simulink model "RigidArmModel_2D"  (R2019a)
settings: Solver=VariableStepAuto  StartTime=0.0  StopTime=stopTime  RelTol=1e-3
undefined symbols (not defined in the file): init_theta_1, init_theta_2, init_theta_dot_1, init_theta_dot_2, k1, k2, L1, L2, m1, m2, t1, t2, x_des, y_des
settings Model: Creator=Shaon  LastModifiedBy=Shaon

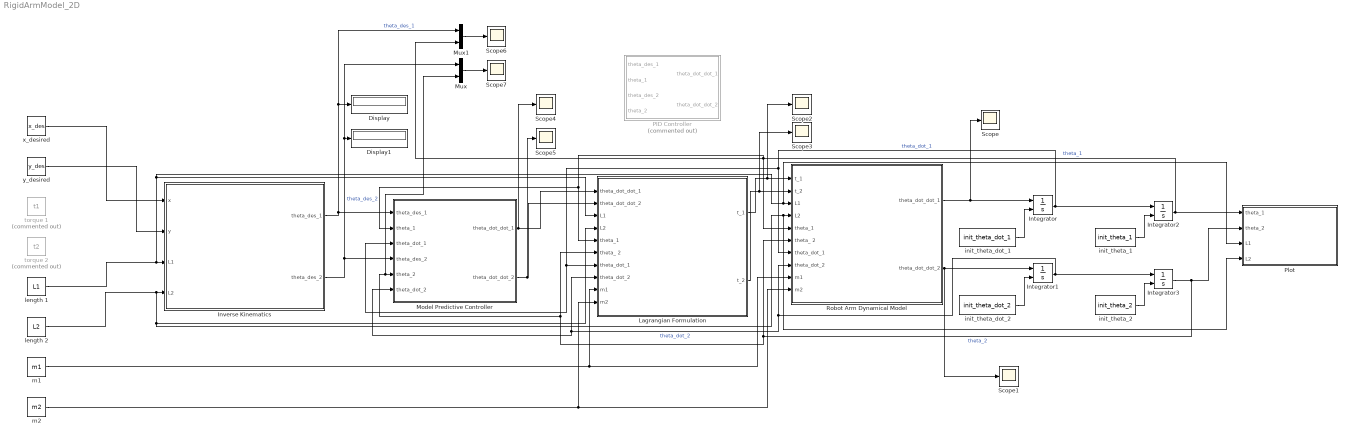
== system RigidArmModel_2D ==
  Display : Display
  Display1 : Display
  Integrator{,1..3} (4 alike) : Integrator  InitialConditionSource=external
  Inverse Kinematics : Subsystem
  Lagrangian Formulation : Subsystem
  Model Predictive Controller : Subsystem
  Mux : Mux  Inputs=2
  Mux1 : Mux  Inputs=2
  PID Controller : Subsystem  Commented=on
  Plot : MATLAB Function  TreatAsAtomicUnit=on
  Robot Arm Dynamical Model : Subsystem
  Scope{,1..7} (8 alike) : Scope
  init_theta_1 : Constant  Value=init_theta_1
  init_theta_2 : Constant  Value=init_theta_2
  init_theta_dot_1 : Constant  Value=init_theta_dot_1
  init_theta_dot_2 : Constant  Value=init_theta_dot_2
  length 1 : Constant  Value=L1
  length 2 : Constant  Value=L2
  m1 : Constant  Value=m1
  m2 : Constant  Value=m2
  torque 1 : Constant  Commented=on  Value=t1
  torque 2 : Constant  Commented=on  Value=t2
  x_desired : Constant  Value=x_des
  y_desired : Constant  Value=y_des
  wires:
  Robot Arm Dynamical Model/1(theta_dot_dot_1) -> Scope/1, Integrator/1
  Robot Arm Dynamical Model/2(theta_dot_dot_2) -> Integrator1/1, Scope1/1
  Integrator/1 -> Robot Arm Dynamical Model/7(theta_dot_1), Model Predictive Controller/3(theta_dot_1), Lagrangian Formulation/7(theta_dot_1), Integrator2/1  "theta_dot_1"
  Integrator1/1 -> Lagrangian Formulation/8(theta_dot_2), Model Predictive Controller/6(theta_dot_2), Robot Arm Dynamical Model/8(theta_dot_2), Integrator3/1  "theta_dot_2"
  Integrator2/1 -> Robot Arm Dynamical Model/5("theta_1 "), Lagrangian Formulation/5("theta_1 "), Model Predictive Controller/2(theta_1), Mux1/2, Plot/1(theta_1)  "theta_1"
  Integrator3/1 -> Lagrangian Formulation/6(theta_ 2), Mux/2, Model Predictive Controller/5(theta_2), Robot Arm Dynamical Model/6(theta_ 2), Plot/2(theta_2)  "theta_2"
  init_theta_1/1 -> Integrator2/2
  init_theta_2/1 -> Integrator3/2
  init_theta_dot_1/1 -> Integrator/2
  init_theta_dot_2/1 -> Integrator1/2
  Inverse Kinematics/1(theta_des_1) -> Model Predictive Controller/1(theta_des_1), Mux1/1, Display/1  "theta_des_1"
  Inverse Kinematics/2(theta_des_2) -> Model Predictive Controller/4(theta_des_2), Mux/1, Display1/1  "theta_des_2"
  x_desired/1 -> Inverse Kinematics/1(x)
  y_desired/1 -> Inverse Kinematics/2(y)
  length 1/1 -> Lagrangian Formulation/3(L1), Plot/3(L1), Robot Arm Dynamical Model/3(L1), Inverse Kinematics/3(L1)
  length 2/1 -> Lagrangian Formulation/4(L2), Plot/4(L2), Robot Arm Dynamical Model/4(L2), Inverse Kinematics/4(L2)
  Lagrangian Formulation/1(t_1) -> Robot Arm Dynamical Model/1(t_1), Scope2/1
  Lagrangian Formulation/2(t_2) -> Robot Arm Dynamical Model/2(t_2), Scope3/1
  m1/1 -> Lagrangian Formulation/9(m1), Robot Arm Dynamical Model/9(m1)
  m2/1 -> Lagrangian Formulation/10(m2), Robot Arm Dynamical Model/10(m2)
  Mux/1 -> Scope7/1
  Mux1/1 -> Scope6/1
  Model Predictive Controller/1(theta_dot_dot_1) -> Scope4/1, Lagrangian Formulation/1(theta_dot_dot_1)
  Model Predictive Controller/2(theta_dot_dot_2) -> Scope5/1, Lagrangian Formulation/2(theta_dot_dot_2)

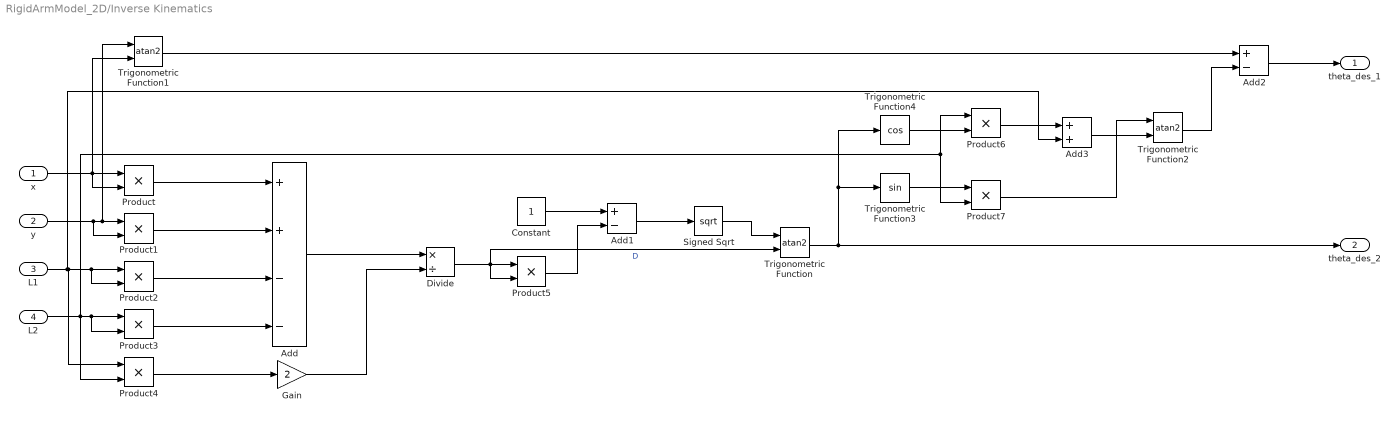
== system RigidArmModel_2D/Inverse Kinematics ==
  x : Inport
  y : Inport  Port=2
  L1 : Inport  Port=3
  L2 : Inport  Port=4
  Add : Sum  Inputs=++--
  Add1 : Sum  Inputs=+-
  Add2 : Sum  Inputs=+-
  Add3 : Sum
  Constant : Constant
  Divide : Product  Inputs=*/
  Gain : Gain  Gain=2
  Product{,1..7} (8 alike) : Product
  Signed Sqrt : Sqrt  SaturateOnIntegerOverflow=on
  Trigonometric Function : Trigonometry  Operator=atan2
  Trigonometric Function1 : Trigonometry  Operator=atan2
  Trigonometric Function2 : Trigonometry  Operator=atan2
  Trigonometric Function3 : Trigonometry
  Trigonometric Function4 : Trigonometry  Operator=cos
  theta_des_1 : Outport
  theta_des_2 : Outport  Port=2
  wires:
  Trigonometric Function2/1 -> Add2/2
  Trigonometric Function/1 -> theta_des_2/1, Trigonometric Function4/1, Trigonometric Function3/1
  Product1/1 -> Add/2
  Product/1 -> Add/1
  Trigonometric Function3/1 -> Product7/1
  y/1 -> Product1/1, Trigonometric Function1/1, Product1/2
  L2/1 -> Product6/1, Product7/2, Product4/2, Product3/2, Product3/1
  Trigonometric Function1/1 -> Add2/1
  Product6/1 -> Add3/1
  Trigonometric Function4/1 -> Product6/2
  Add2/1 -> theta_des_1/1
  Add3/1 -> Trigonometric Function2/2
  Constant/1 -> Add1/1
  L1/1 -> Add3/2, Product4/1, Product2/2, Product2/1
  Signed Sqrt/1 -> Trigonometric Function/1
  Add/1 -> Divide/1
  Product7/1 -> Trigonometric Function2/1
  x/1 -> Product/2, Product/1, Trigonometric Function1/2
  Product5/1 -> Add1/2
  Product2/1 -> Add/3
  Add1/1 -> Signed Sqrt/1
  Divide/1 -> Product5/2, Product5/1, Trigonometric Function/2  "D"
  Gain/1 -> Divide/2
  Product4/1 -> Gain/1
  Product3/1 -> Add/4

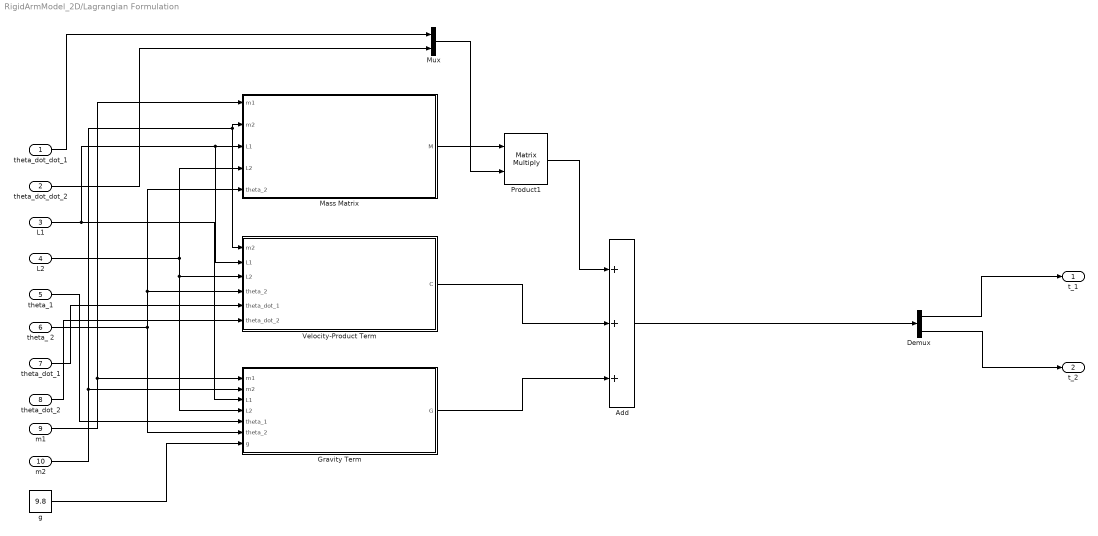
== system RigidArmModel_2D/Lagrangian Formulation ==
  theta_dot_dot_1 : Inport
  theta_dot_dot_2 : Inport  Port=2
  L1 : Inport  Port=3
  L2 : Inport  Port=4
  "theta_1 " : Inport  Port=5
  theta_ 2 : Inport  Port=6
  theta_dot_1 : Inport  Port=7
  theta_dot_2 : Inport  Port=8
  m1 : Inport  Port=9
  m2 : Inport  Port=10
  Add : Sum  Inputs=+++
  Demux : Demux  Outputs=2
  Gravity Term : MATLAB Function  TreatAsAtomicUnit=on
  Mass Matrix : MATLAB Function  TreatAsAtomicUnit=on
  Mux : Mux  Inputs=2
  Product1 : Product  Multiplication=Matrix(*)
  Velocity-Product Term : MATLAB Function  TreatAsAtomicUnit=on
  g : Constant  Value=9.8
  t_1 : Outport
  t_2 : Outport  Port=2
  wires:
  Velocity-Product Term/1(C) -> Add/2
  Gravity Term/1(G) -> Add/3
  Add/1 -> Demux/1
  Demux/1 -> t_1/1
  Demux/2 -> t_2/1
  theta_dot_dot_1/1 -> Mux/1
  theta_dot_dot_2/1 -> Mux/2
  m1/1 -> Gravity Term/1(m1), Mass Matrix/1(m1)
  m2/1 -> Gravity Term/2(m2), Velocity-Product Term/1(m2), Mass Matrix/2(m2)
  L1/1 -> Gravity Term/3(L1), Mass Matrix/3(L1), Velocity-Product Term/2(L1)
  L2/1 -> Velocity-Product Term/3(L2), Gravity Term/4(L2), Mass Matrix/4(L2)
  theta_ 2/1 -> Gravity Term/6(theta_2), Velocity-Product Term/4(theta_2), Mass Matrix/5(theta_2)
  theta_dot_1/1 -> Velocity-Product Term/5(theta_dot_1)
  theta_dot_2/1 -> Velocity-Product Term/6(theta_dot_2)
  "theta_1 "/1 -> Gravity Term/5(theta_1)
  g/1 -> Gravity Term/7(g)
  Mass Matrix/1(M) -> Product1/1
  Mux/1 -> Product1/2
  Product1/1 -> Add/1

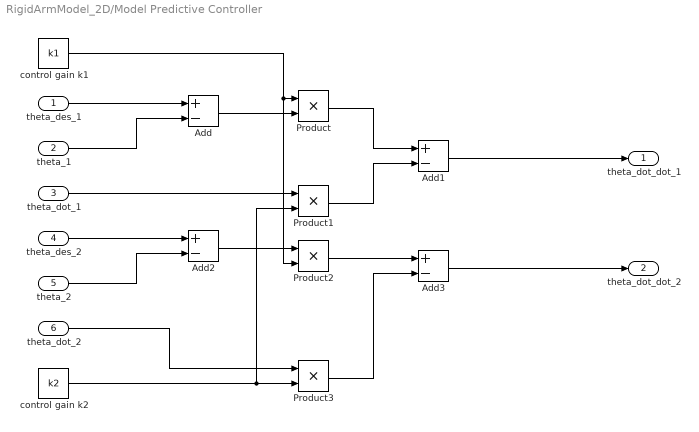
== system RigidArmModel_2D/Model Predictive Controller ==
  theta_des_1 : Inport
  theta_1 : Inport  Port=2
  theta_dot_1 : Inport  Port=3
  theta_des_2 : Inport  Port=4
  theta_2 : Inport  Port=5
  theta_dot_2 : Inport  Port=6
  Add{,1..3} (4 alike) : Sum  Inputs=+-
  Product{,1..3} (4 alike) : Product
  control gain k1 : Constant  Value=k1
  control gain k2 : Constant  Value=k2
  theta_dot_dot_1 : Outport
  theta_dot_dot_2 : Outport  Port=2
  wires:
  control gain k1/1 -> Product2/2, Product/1
  Product1/1 -> Add1/2
  Product3/1 -> Add3/2
  Add1/1 -> theta_dot_dot_1/1
  Add2/1 -> Product2/1
  Product/1 -> Add1/1
  theta_dot_2/1 -> Product3/1
  Add3/1 -> theta_dot_dot_2/1
  control gain k2/1 -> Product3/2, Product1/2
  Product2/1 -> Add3/1
  theta_2/1 -> Add2/2
  theta_dot_1/1 -> Product1/1
  theta_des_1/1 -> Add/1
  Add/1 -> Product/2
  theta_1/1 -> Add/2
  theta_des_2/1 -> Add2/1

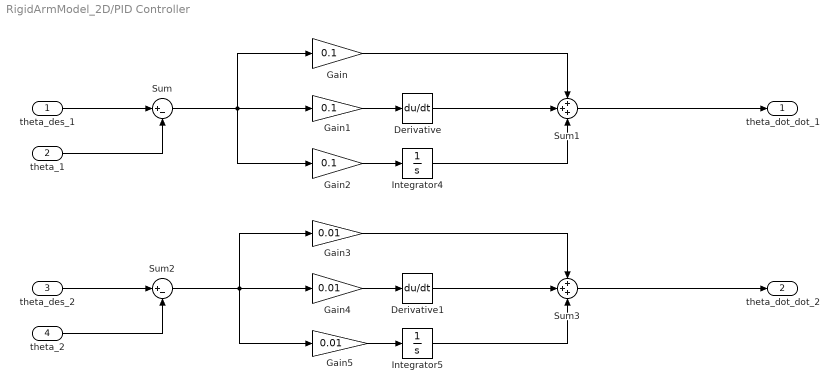
== system RigidArmModel_2D/PID Controller ==
  theta_des_1 : Inport
  theta_1 : Inport  Port=2
  theta_des_2 : Inport  Port=3
  theta_2 : Inport  Port=4
  Derivative : Derivative
  Derivative1 : Derivative
  Gain : Gain  Gain=0.1
  Gain1 : Gain  Gain=0.1
  Gain2 : Gain  Gain=0.1
  Gain3 : Gain  Gain=0.01
  Gain4 : Gain  Gain=0.01
  Gain5 : Gain  Gain=0.01
  Integrator4 : Integrator
  Integrator5 : Integrator
  Sum : Sum  Inputs=|+-
  Sum1 : Sum  Inputs=+++
  Sum2 : Sum  Inputs=|+-
  Sum3 : Sum  Inputs=+++
  theta_dot_dot_1 : Outport
  theta_dot_dot_2 : Outport  Port=2
  wires:
  Integrator5/1 -> Sum3/3
  Sum3/1 -> theta_dot_dot_2/1
  Gain3/1 -> Sum3/1
  Gain4/1 -> Derivative1/1
  Derivative1/1 -> Sum3/2
  Gain5/1 -> Integrator5/1
  theta_des_2/1 -> Sum2/1
  Gain/1 -> Sum1/1
  theta_1/1 -> Sum/2
  Derivative/1 -> Sum1/2
  theta_2/1 -> Sum2/2
  Gain1/1 -> Derivative/1
  Gain2/1 -> Integrator4/1
  Sum1/1 -> theta_dot_dot_1/1
  Integrator4/1 -> Sum1/3
  theta_des_1/1 -> Sum/1
  Sum/1 -> Gain2/1, Gain/1, Gain1/1
  Sum2/1 -> Gain3/1, Gain5/1, Gain4/1

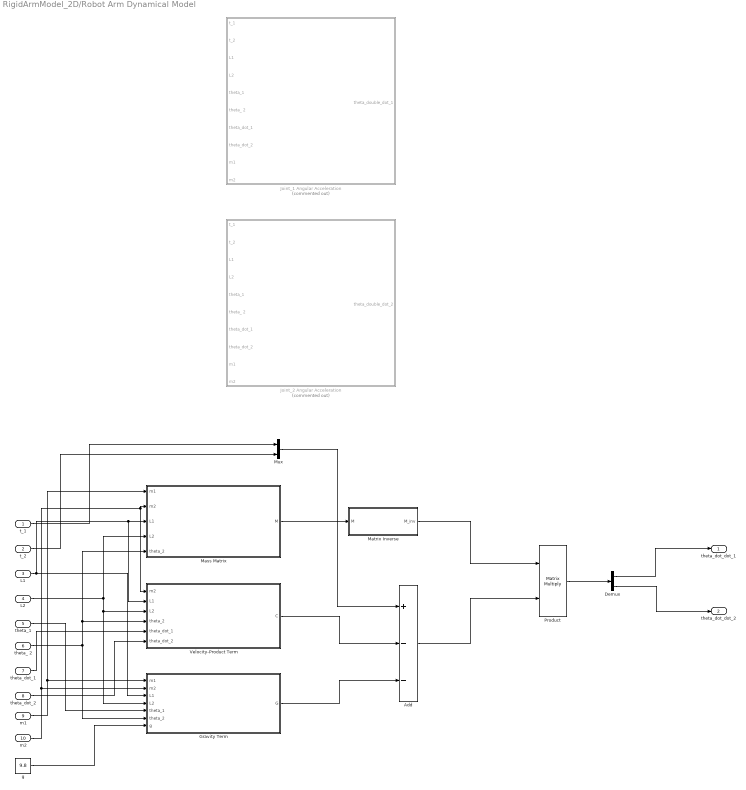
== system RigidArmModel_2D/Robot Arm Dynamical Model ==
  t_1 : Inport
  t_2 : Inport  Port=2
  L1 : Inport  Port=3
  L2 : Inport  Port=4
  "theta_1 " : Inport  Port=5
  theta_ 2 : Inport  Port=6
  theta_dot_1 : Inport  Port=7
  theta_dot_2 : Inport  Port=8
  m1 : Inport  Port=9
  m2 : Inport  Port=10
  Add : Sum  Inputs=+--
  Demux : Demux  Outputs=2
  Gravity Term : MATLAB Function  TreatAsAtomicUnit=on
  Joint_1 Angular Acceleration : Subsystem  Commented=on
  Joint_2 Angular Acceleration : Subsystem  Commented=on
  Mass Matrix : MATLAB Function  TreatAsAtomicUnit=on
  Matrix Inverse : MATLAB Function  TreatAsAtomicUnit=on
  Mux : Mux  Inputs=2
  Product : Product  Multiplication=Matrix(*)
  Velocity-Product Term : MATLAB Function  TreatAsAtomicUnit=on
  g : Constant  Value=9.8
  theta_dot_dot_1 : Outport
  theta_dot_dot_2 : Outport  Port=2
  wires:
  Mux/1 -> Add/1
  Velocity-Product Term/1(C) -> Add/2
  Gravity Term/1(G) -> Add/3
  Mass Matrix/1(M) -> Matrix Inverse/1(M)
  Matrix Inverse/1(M_inv) -> Product/1
  Add/1 -> Product/2
  Product/1 -> Demux/1
  Demux/1 -> theta_dot_dot_1/1
  Demux/2 -> theta_dot_dot_2/1
  t_1/1 -> Mux/1
  t_2/1 -> Mux/2
  m1/1 -> Gravity Term/1(m1), Mass Matrix/1(m1)
  m2/1 -> Gravity Term/2(m2), Velocity-Product Term/1(m2), Mass Matrix/2(m2)
  L1/1 -> Gravity Term/3(L1), Mass Matrix/3(L1), Velocity-Product Term/2(L1)
  L2/1 -> Velocity-Product Term/3(L2), Gravity Term/4(L2), Mass Matrix/4(L2)
  theta_ 2/1 -> Gravity Term/6(theta_2), Velocity-Product Term/4(theta_2), Mass Matrix/5(theta_2)
  theta_dot_1/1 -> Velocity-Product Term/5(theta_dot_1)
  theta_dot_2/1 -> Velocity-Product Term/6(theta_dot_2)
  "theta_1 "/1 -> Gravity Term/5(theta_1)
  g/1 -> Gravity Term/7(g)

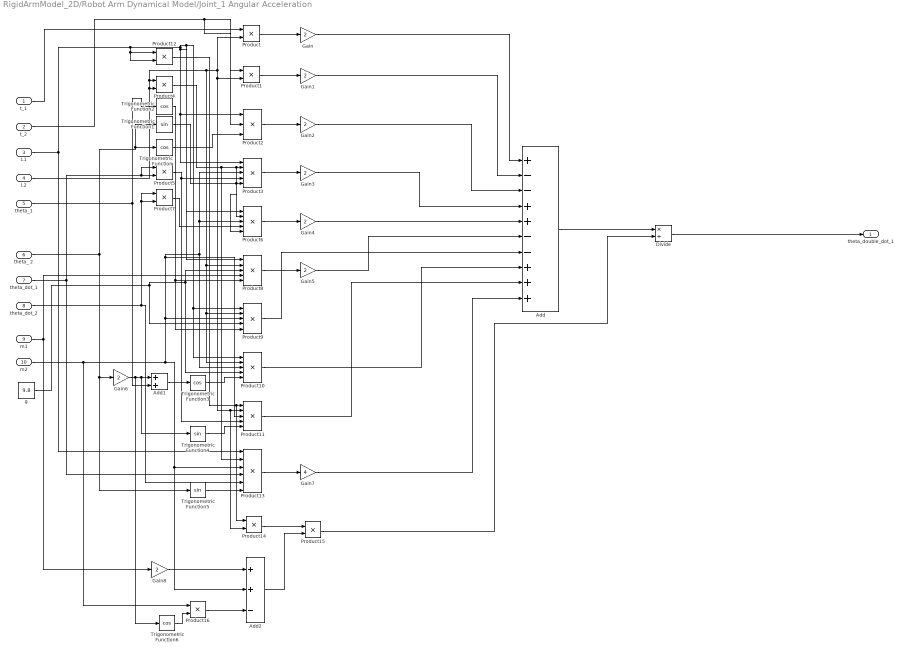
== system RigidArmModel_2D/Robot Arm Dynamical Model/Joint_1 Angular Acceleration ==
  t_1 : Inport
  t_2 : Inport  Port=2
  L1 : Inport  Port=3
  L2 : Inport  Port=4
  "theta_1 " : Inport  Port=5
  theta_ 2 : Inport  Port=6
  theta_dot_1 : Inport  Port=7
  theta_dot_2 : Inport  Port=8
  m1 : Inport  Port=9
  m2 : Inport  Port=10
  Add : Sum  Inputs=+--++--+++
  Add1 : Sum
  Add2 : Sum  Inputs=++-
  Divide : Product  Inputs=*/
  Gain{,1..6,8} (8 alike) : Gain  Gain=2
  Gain7 : Gain  Gain=4
  Product{,1,4..5,7,12,14..16} (9 alike) : Product
  Product{3,6,8..11} (6 alike) : Product  Inputs=5
  Product13 : Product  Inputs=6
  Product2 : Product  Inputs=3
  Trigonometric Function{,2..3,6} (4 alike) : Trigonometry  Operator=cos
  Trigonometric Function1 : Trigonometry
  Trigonometric Function4 : Trigonometry
  Trigonometric Function5 : Trigonometry
  g : Constant  Value=9.8
  theta_double_dot_1 : Outport
  wires:
  Product15/1 -> Divide/2
  theta_dot_1/1 -> Product13/4, Product5/1, Product5/2
  theta_dot_2/1 -> Product13/5, Product7/1, Product7/2
  Product11/1 -> Add/9
  Trigonometric Function1/1 -> Product6/5, Product3/5
  Trigonometric Function6/1 -> Product16/2
  Product7/1 -> Product6/4
  Product2/1 -> Gain2/1
  g/1 -> Product10/4, Product8/3, Product9/4
  Product8/1 -> Gain5/1
  Product1/1 -> Gain1/1
  Product4/1 -> Product6/2, Product3/2, Product13/2
  m2/1 -> Product16/1, Product13/3, Add2/2, Product11/3, Product10/3, Product6/3, Product3/3, Product9/3
  L1/1 -> Product13/1, Product12/2, Product12/1, Product10/1, Product9/1, Product6/1, Product8/1, Product3/1, Product2/1
  t_1/1 -> Product/1
  "theta_1 "/1 -> Trigonometric Function2/1, Add1/2
  Gain5/1 -> Add/6
  L2/1 -> Product10/2, Product9/2, Product8/2, Product1/2, Product11/2, Product14/2, Product/2, Product4/1, Product4/2
  Gain/1 -> Add/1
  Product3/1 -> Gain3/1
  t_2/1 -> Product2/2, Product1/1
  Product12/1 -> Product14/1, Product11/1
  Gain1/1 -> Add/2
  Product6/1 -> Gain4/1
  Product/1 -> Gain/1
  Add/1 -> Divide/1
  Product13/1 -> Gain7/1
  Gain8/1 -> Add2/1
  Trigonometric Function2/1 -> Product9/5, Product8/5
  Gain6/1 -> Trigonometric Function4/1, Add1/1, Trigonometric Function6/1
  Trigonometric Function/1 -> Product2/3
  theta_ 2/1 -> Trigonometric Function5/1, Gain6/1, Trigonometric Function1/1, Trigonometric Function/1
  Gain4/1 -> Add/5
  Product10/1 -> Add/8
  Gain3/1 -> Add/4
  m1/1 -> Gain8/1, Product8/4
  Product16/1 -> Add2/3
  Add1/1 -> Trigonometric Function3/1
  Trigonometric Function3/1 -> Product10/5
  Product9/1 -> Add/7
  Product14/1 -> Product15/1
  Product5/1 -> Product11/4, Product3/4
  Gain2/1 -> Add/3
  Trigonometric Function4/1 -> Product11/5
  Trigonometric Function5/1 -> Product13/6
  Add2/1 -> Product15/2
  Gain7/1 -> Add/10
  Divide/1 -> theta_double_dot_1/1

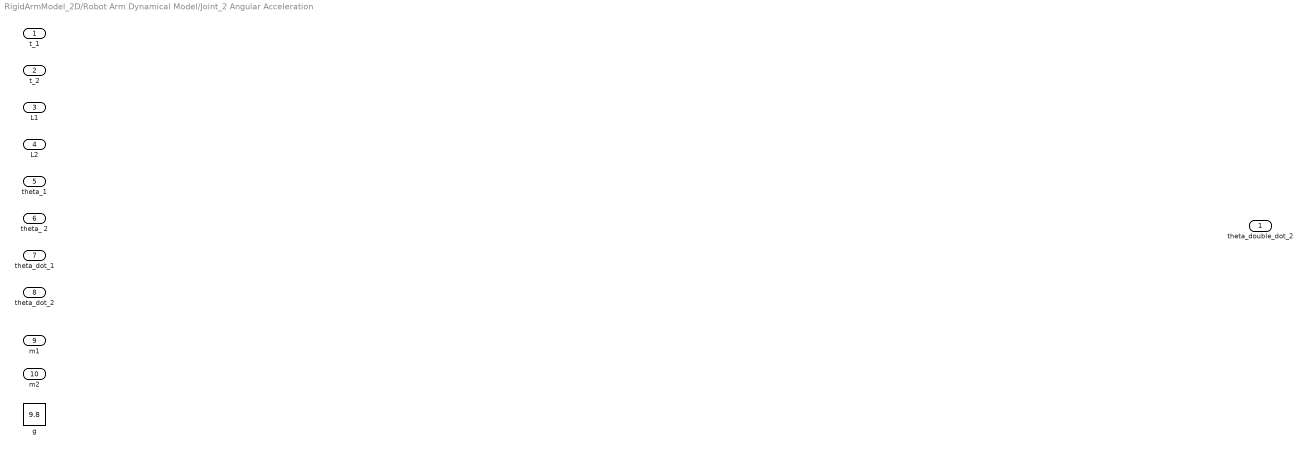
== system RigidArmModel_2D/Robot Arm Dynamical Model/Joint_2 Angular Acceleration ==
  t_1 : Inport
  t_2 : Inport  Port=2
  L1 : Inport  Port=3
  L2 : Inport  Port=4
  "theta_1 " : Inport  Port=5
  theta_ 2 : Inport  Port=6
  theta_dot_1 : Inport  Port=7
  theta_dot_2 : Inport  Port=8
  m1 : Inport  Port=9
  m2 : Inport  Port=10
  g : Constant  Value=9.8
  theta_double_dot_2 : Outport

== matlab function RigidArmModel_2D/Robot Arm Dynamical Model/Velocity-Product Term ==
  data: m2 input; C output size=[2,1]; L1 input; L2 input; theta_2 input; theta_dot_1 input; theta_dot_2 input
function C = velocity_product(m2, L1, L2, theta_2, theta_dot_1, theta_dot_2)
    %#codegen
    C_11 = -m2 * L1 * L2 * sin(theta_2) * (2 * theta_dot_1 * theta_dot_2 + theta_dot_2^2);
    C_21 = m2 * L1 * L2 * theta_dot_1^2 * sin(theta_2);
    C = [C_11; C_21];
end

== matlab function RigidArmModel_2D/Robot Arm Dynamical Model/Mass Matrix ==
  data: m1 input; M output size=[2,2]; m2 input; L1 input; L2 input; theta_2 input
function M = mass_matrix(m1, m2, L1, L2,theta_2)
    %#codegen
    M_11 = m1 * L1^2 + m2 * (L1^2 + 2 * L1 * L2 * cos(theta_2) + L2^2);
    M_12 = m2 * (L1 * L2 * cos(theta_2) + L2^2);
    M_21 = m2 * (L1 * L2 * cos(theta_2) + L2^2);
    M_22 = m2 * L2^2;
    M = [M_11 M_12; M_21 M_22];
end

== matlab function RigidArmModel_2D/Robot Arm Dynamical Model/Gravity Term ==
  data: m1 input; G output size=[2,1]; m2 input; L1 input; L2 input; theta_1 input; theta_2 input; g input
function G = gravity(m1, m2, L1, L2, theta_1, theta_2, g)
    %#codegen
    G_11 = (m1 + m2) * L1 * g * cos(theta_1) + m2 * g * L2 * cos(theta_1 + theta_2);
    G_21 = m2 * g * L2 * cos(theta_1 + theta_2);
    G = [G_11; G_21];
end

== matlab function RigidArmModel_2D/Robot Arm Dynamical Model/Matrix Inverse ==
  data: M input size=[2,2]; M_inv output size=[2,2]
function M_inv = matrix_inv(M)
    M_inv = inv(M);
end

== matlab function RigidArmModel_2D/Plot ==
  data: theta_1 input; theta_2 input; L1 input; L2 input
function create_plot(theta_1, theta_2, L1, L2)
    coder.extrinsic('plot');

    x0 = 0;
    y0 = 0;
    x1 = L1 * cos(theta_1);
    y1 = L1 * sin(theta_1);
    x2 = L1 * cos(theta_1) + L2 * cos(theta_1 + theta_2);
    y2 = L1 * sin(theta_1) + L2 * sin(theta_1 + theta_2);
    
    clf;
    plot(0, 0, 's', 'MarkerFaceColor', 'red');
    hold on
    plot(x1, y1, 'o', 'MarkerFaceColor', 'green');
    hold on
    plot([x0 x1 x2], [y0 y1 y2]);
    
%     plot([x0 x1 x2], [y0 y1 y2], '-o', 'MarkerFaceColor', 'red');
    xlim([-2 2]);
    ylim([-2 2]);
    axis('equal');
end

== matlab function RigidArmModel_2D/Lagrangian Formulation/Gravity Term ==
  data: m1 input; G output size=[2,1]; m2 input; L1 input; L2 input; theta_1 input; theta_2 input; g input
function G = gravity(m1, m2, L1, L2, theta_1, theta_2, g)
    %#codegen
    G_11 = (m1 + m2) * L1 * g * cos(theta_1) + m2 * g * L2 * cos(theta_1 + theta_2);
    G_21 = m2 * g * L2 * cos(theta_1 + theta_2);
    G = [G_11; G_21];
end

== matlab function RigidArmModel_2D/Lagrangian Formulation/Mass Matrix ==
  data: m1 input; M output size=[2,2]; m2 input; L1 input; L2 input; theta_2 input
function M = mass_matrix(m1, m2, L1, L2,theta_2)
    %#codegen
    M_11 = m1 * L1^2 + m2 * (L1^2 + 2 * L1 * L2 * cos(theta_2) + L2^2);
    M_12 = m2 * (L1 * L2 * cos(theta_2) + L2^2);
    M_21 = m2 * (L1 * L2 * cos(theta_2) + L2^2);
    M_22 = m2 * L2^2;
    M = [M_11 M_12; M_21 M_22];
end

== matlab function RigidArmModel_2D/Lagrangian Formulation/Velocity-Product Term ==
  data: m2 input; C output size=[2,1]; L1 input; L2 input; theta_2 input; theta_dot_1 input; theta_dot_2 input
function C = velocity_product(m2, L1, L2, theta_2, theta_dot_1, theta_dot_2)
    %#codegen
    C_11 = -m2 * L1 * L2 * sin(theta_2) * (2 * theta_dot_1 * theta_dot_2 + theta_dot_2^2);
    C_21 = m2 * L1 * L2 * theta_dot_1^2 * sin(theta_2);
    C = [C_11; C_21];
end
